simulink model "GA_test_x"  (R2022a)
settings: Solver=VariableStepAuto  StartTime=0.0  StopTime=10.0  RelTol=1e-3
values from neighbouring files (symbols this model uses):
  fs = 30000    [ga_5.mat]    (also in ga_6.mat; ga_ok_1.mat; ga_ok_10.mat; ga_ok_2.mat)
  Gv = 15    [ga_5.mat]    (also in ga_6.mat; ga_ok_1.mat; ga_ok_10.mat; ga_ok_2.mat)
  R = conv(Hr, [parms(1) parms(2)])    [controller_test.m]    (also in controller_test_ok_10.m; controller_test_ok_3.m; controller_test_ok_6.m; controller_test_ok_7.m)
  S = conv(Hs, [1 parms(3) parms(4)])    [controller_test.m]    (also in controller_test_ok_10.m; controller_test_ok_3.m; controller_test_ok_6.m; controller_test_ok_7.m)
  wv = 4000    [ga_5.mat]    (also in ga_6.mat; ga_ok_1.mat; ga_ok_10.mat; ga_ok_2.mat)
undefined symbols (not defined in the file or in its folder): Gax, Gcs, wax, wcs, zetax
libraries: simulink x1, spsTriangleGeneratorLib x1
settings Model: Creator=doamarar  LastModifiedBy=doamarar

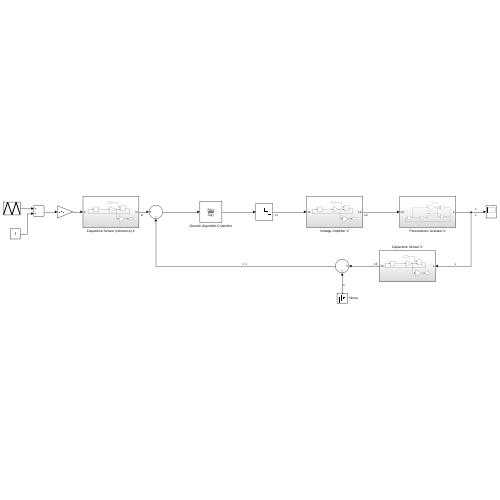
[thumbnail: Simulink's stored preview of the top-level diagram]
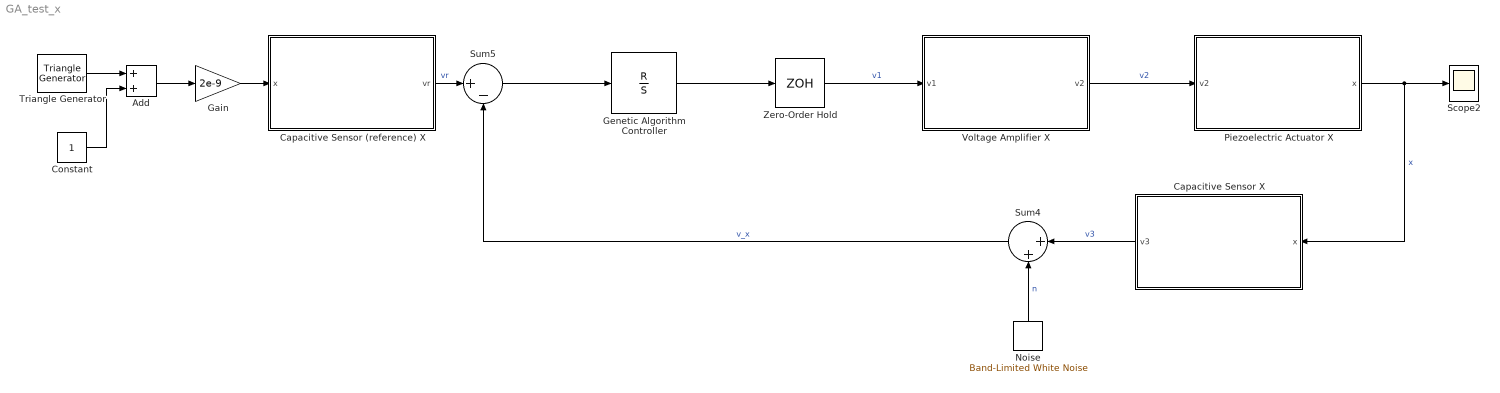
== system GA_test_x ==
  Add : Sum
  Capacitive Sensor (reference) X : Subsystem
  Capacitive Sensor X : Subsystem
  Constant : Constant
  Gain : Gain  Gain=2e-9
  Genetic Algorithm Controller : DiscreteFilter  Numerator=R  Denominator=S  SampleTime=1/fs
  Noise : simulink/Sources/Band-Limited White Noise  Cov=[0.00000000000000001]  Ts=5e-5  seed=[23341]
  Piezoelectric Actuator X : Subsystem
  Scope2 : Scope
  Sum4 : Sum  Inputs=|++
  Sum5 : Sum  Inputs=|+-
  Triangle Generator : spsTriangleGeneratorLib/Triangle Generator  Freq=5  Phase=0  Ts=5e-5
  Voltage Amplifier X : Subsystem
  Zero-Order Hold : ZeroOrderHold  SampleTime=5e-5
  wires:
  Constant/1 -> Add/2
  Noise/1 -> Sum4/2  "n"
  Sum4/1 -> Sum5/2  "v_x"
  Gain/1 -> Capacitive Sensor (reference) X/1(x)
  Triangle Generator/1 -> Add/1
  Add/1 -> Gain/1
  Capacitive Sensor X/1(v3) -> Sum4/1  "v3"
  Capacitive Sensor (reference) X/1(vr) -> Sum5/1  "vr"
  Zero-Order Hold/1 -> Voltage Amplifier X/1(v1)  "v1"
  Piezoelectric Actuator X/1(x) -> Scope2/1, Capacitive Sensor X/1(x)  "x"
  Voltage Amplifier X/1(v2) -> Piezoelectric Actuator X/1(v2)  "v2"
  Sum5/1 -> Genetic Algorithm Controller/1
  Genetic Algorithm Controller/1 -> Zero-Order Hold/1

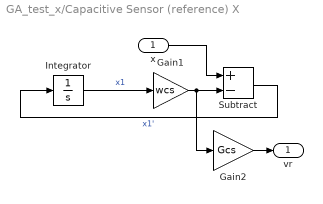
== system GA_test_x/Capacitive Sensor (reference) X ==
  x : Inport
  Gain1 : Gain  Gain=wcs
  Gain2 : Gain  Gain=Gcs
  Integrator : Integrator
  Subtract : Sum  Inputs=+-
  vr : Outport
  wires:
  x/1 -> Subtract/1
  Gain2/1 -> vr/1
  Gain1/1 -> Subtract/2, Gain2/1
  Subtract/1 -> Integrator/1  "x1'"
  Integrator/1 -> Gain1/1  "x1"

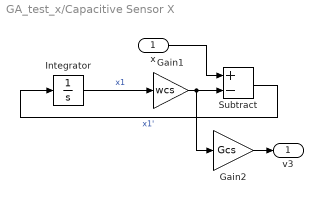
== system GA_test_x/Capacitive Sensor X ==
  x : Inport
  Gain1 : Gain  Gain=wcs
  Gain2 : Gain  Gain=Gcs
  Integrator : Integrator
  Subtract : Sum  Inputs=+-
  v3 : Outport
  wires:
  x/1 -> Subtract/1
  Gain2/1 -> v3/1
  Gain1/1 -> Subtract/2, Gain2/1
  Subtract/1 -> Integrator/1  "x1'"
  Integrator/1 -> Gain1/1  "x1"

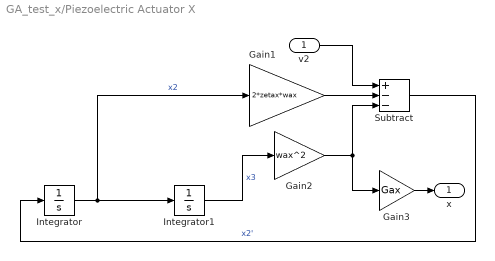
== system GA_test_x/Piezoelectric Actuator X ==
  v2 : Inport
  Gain1 : Gain  Gain=2*zetax*wax
  Gain2 : Gain  Gain=wax^2
  Gain3 : Gain  Gain=Gax
  Integrator : Integrator
  Integrator1 : Integrator
  Subtract : Sum  Inputs=+--
  x : Outport
  wires:
  Integrator1/1 -> Gain2/1  "x3"
  Gain3/1 -> x/1
  Integrator/1 -> Integrator1/1, Gain1/1  "x2"
  Gain2/1 -> Gain3/1, Subtract/3
  v2/1 -> Subtract/1
  Gain1/1 -> Subtract/2
  Subtract/1 -> Integrator/1  "x2'"

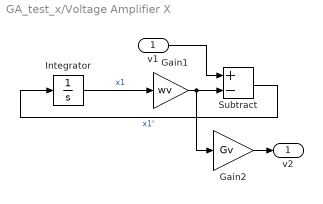
== system GA_test_x/Voltage Amplifier X ==
  v1 : Inport
  Gain1 : Gain  Gain=wv
  Gain2 : Gain  Gain=Gv
  Integrator : Integrator
  Subtract : Sum  Inputs=+-
  v2 : Outport
  wires:
  v1/1 -> Subtract/1
  Gain2/1 -> v2/1
  Gain1/1 -> Subtract/2, Gain2/1
  Subtract/1 -> Integrator/1  "x1'"
  Integrator/1 -> Gain1/1  "x1"
